simulink model "forced_choice"  (Simulink 6.6)
settings: Solver=FixedStepDiscrete  StartTime=0.0  StopTime=Inf  FixedStep=.001  RelTol=1e-3
undefined symbols (not defined in the file or in its folder): dfilt
libraries: xpclib x12, limblab x7, simulink x6, xpcnilib x4, dsparch4 x4, xpcmeasurementcomputinglib x2
CloseFcn:
  | rtwprivate ssgencode ModelCloseRequest rwalk_multi_local_v1
settings Model: Creator=limblab  LastModifiedBy=limblab  ExtModeArmWhenConnect=off  BufferReuse=off
settings DataIOCC: LimitDataPoints=off  SaveFormat=StructureWithTime  SaveState=on  SignalLoggingName=sigsOut
settings OptimizationCC: BlockReduction=off  BooleanDataType=off  OptimizeBlockIOStorage=off  BufferReuse=off  EnforceIntegerDowncast=off  ExpressionFolding=off  FoldNonRolledExpr=off  LocalBlockOutputs=off
settings DebuggingCC: SignalResolutionControl=TryResolveAllWithWarning  SolverPrmCheckMsg=none  MultiTaskDSMMsg=warning  MultiTaskCondExecSysMsg=none  StrictBusMsg=None
settings HardwareCC: TargetIntDivRoundTo=Floor  TargetEndianess=LittleEndian  TargetHWDeviceType=32-bit xPC Target (Intel Pentium)
settings RTWCC: SystemTargetFile=xpctarget.tlc  TemplateMakefile=xpc_default_tmf  Description=xPC Target  GenerateReport=on  ProcessScript=xpctarget_make_rtw_hook  IncludeERTFirstTime=on
settings xpcTargetCC: TargetFcnLib=ansi_tfl_tmw.mat  GenFloatMathFcnCalls=ANSI_C  PortableWordSizes=off

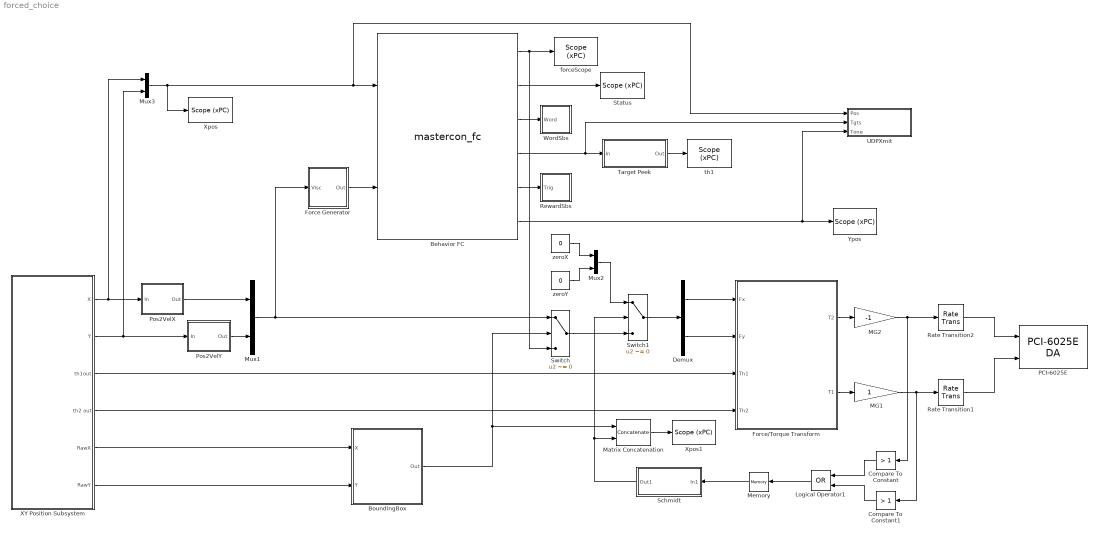
== system forced_choice ==
  Behavior FC : S-Function  FunctionName=mastercon_fc  Parameters=3 0 1 .5 1 .5 1 10 3 3 10
      mask Display:
      | disp('Master Control\nForced-Choice')
      | port_label('input',1,'pos')
      | port_label('input',2,'force')
      | port_label('output',1,'force')
      | port_label('output',2,'status')
      | port_label('output',3,'word')
      | port_label('output',4,'targets')
      | port_label('output',5,'reward')
      | port_label('output',6,'tone')
  BoundingBox : Subsystem
  Compare To Constant : simulink/Logic and Bit Operations/Compare To Constant  Orientation=left  SystemSampleTime=-1  relop=>  const=1  LogicOutDataTypeMode=uint8  ZeroCross=off
  Compare To Constant1 : simulink/Logic and Bit Operations/Compare To Constant  Orientation=left  SystemSampleTime=-1  relop=>  const=1  LogicOutDataTypeMode=uint8  ZeroCross=off
  Demux : Demux  Outputs=2
  Force Generator : Subsystem
  Force/Torque Transform : Subsystem  TreatAsAtomicUnit=on
      mask Display:
      | port_label('output', 1, 'T2')
      | port_label('output', 2, 'T1')
      | port_label('input', 1, 'Fx')
      | port_label('input', 2, 'Fy')
      | port_label('input', 3, 'Th1')
      | port_label('input', 4, 'Th2')
  Logical Operator1 : Logic  Orientation=left  Operator=OR  AllPortsSameDT=off  OutDataTypeMode=Boolean
  MG1 : Gain
  MG2 : Gain  Gain=-1
  Matrix Concatenation : Concatenate  Mode=Multidimensional array
  Memory : Memory  Orientation=left
  Mux1 : Mux  Inputs=2
  Mux2 : Mux  Inputs=2
  Mux3 : Mux  Inputs=2
  "PCI-6025E " : xpcnilib/D//A/PCI-6025E DA  channel=[1 2]  reset=[1 1]  initValue=[0 0]  sampletime=0.01  slot=[0 18]
  Pos2VelX : Subsystem
  Pos2VelY : Subsystem
  Rate Transition1 : RateTransition
  Rate Transition2 : RateTransition
  RewardSbs : Subsystem
  Schmidt : Subsystem  Orientation=left  mask(Schmidt Trigger){Time=10}
      mask help: Creates an output pulse of the specified time in seconds when trig goes high
      mask Help: Creates an output pulse of the specified time in seconds when trig goes high
      mask Display:
      | port_label('output',1,'out')
      | port_label('input',1,'trig')
      | fprintf('t = %d',Time)
  Status : xpclib/Misc./Scope (xPC)   SystemSampleTime=-1  scopeno=3  scopetype=Target  autostart=on  viewmode=Numerical  formatstr='%2.2f'  grid=on  ylimits=[-10,10]  nosamples=10  noprepostsamples=0  interleave=10  triggermode=FreeRun  triggersignal=1  triggerlevel=0.0  triggerslope=Either  triggerscope=1  triggersample=0  filename=data.dat  mode=Lazy  writesize=512  autorestart=off
  Switch : Switch  Criteria=u2 ~= 0  ZeroCross=off
  Switch1 : Switch  Criteria=u2 ~= 0  ZeroCross=off
  Target Peek : Subsystem
  UDPXmit : Subsystem
  WordSbs : Subsystem
  XY Position Subsystem : Subsystem
  Xpos : xpclib/Misc./Scope (xPC)   SystemSampleTime=-1  scopeno=1  scopetype=Target  autostart=on  viewmode=Numerical  formatstr=['%15.2f' '%15.2f']  grid=on  ylimits=[-10,10]  nosamples=10  noprepostsamples=0  interleave=10  triggermode=FreeRun  triggersignal=1  triggerlevel=0.0  triggerslope=Either  triggerscope=1  triggersample=0  filename=data.dat  mode=Lazy  writesize=512  autorestart=off
  Xpos1 : xpclib/Misc./Scope (xPC)   SystemSampleTime=-1  scopeno=5  scopetype=Target  autostart=on  viewmode=Numerical  formatstr='%15.2f'  grid=on  ylimits=[-10,10]  nosamples=10  noprepostsamples=0  interleave=10  triggermode=FreeRun  triggersignal=1  triggerlevel=0.0  triggerslope=Either  triggerscope=1  triggersample=0  filename=data.dat  mode=Lazy  writesize=512  autorestart=off
  Ypos : xpclib/Misc./Scope (xPC)   SystemSampleTime=-1  scopeno=2  scopetype=Target  autostart=on  viewmode=Numerical  formatstr='%15.2f'  grid=on  ylimits=[-10,10]  nosamples=10  noprepostsamples=0  interleave=10  triggermode=FreeRun  triggersignal=1  triggerlevel=0.0  triggerslope=Either  triggerscope=1  triggersample=0  filename=data.dat  mode=Lazy  writesize=512  autorestart=off
  forceScope : xpclib/Misc./Scope (xPC)   SystemSampleTime=-1  scopeno=7  scopetype=Target  autostart=on  viewmode=Numerical  formatstr='%2.2f'  grid=on  ylimits=[0,0]  nosamples=7  noprepostsamples=0  interleave=1  triggermode=FreeRun  triggersignal=1  triggerlevel=0.0  triggerslope=Either  triggerscope=1  triggersample=0  filename=data.dat  mode=Lazy  writesize=512  autorestart=off
  th1 : xpclib/Misc./Scope (xPC)   SystemSampleTime=-1  scopeno=4  scopetype=Target  autostart=on  viewmode=Numerical  formatstr=['%d' '%2.2f' '%2.2f']  grid=on  ylimits=[0,0]  nosamples=7  noprepostsamples=0  interleave=1  triggermode=FreeRun  triggersignal=1  triggerlevel=0.0  triggerslope=Either  triggerscope=1  triggersample=0  filename=data.dat  mode=Lazy  writesize=512  autorestart=off
  zeroX : Constant  Value=0
  zeroY : Constant  Value=0
  wires:
  XY Position Subsystem/1(X) -> Pos2VelX/1(In), Mux3/1
  XY Position Subsystem/2(Y) -> Pos2VelY/1(In), Mux3/2
  MG2/1 -> Rate Transition2/1, Compare To Constant/1
  MG1/1 -> Rate Transition1/1, Compare To Constant1/1
  Force/Torque Transform/1(T2) -> MG2/1
  Force/Torque Transform/2("T1 ") -> MG1/1
  XY Position Subsystem/3(th1out) -> Force/Torque Transform/3(Th1)
  XY Position Subsystem/4(th2 out) -> Force/Torque Transform/4(Th2)
  Demux/1 -> Force/Torque Transform/1(Fx)
  Demux/2 -> Force/Torque Transform/2(Fy)
  Mux1/1 -> Switch/1, Force Generator/1(Visc)
  XY Position Subsystem/5(RawX) -> BoundingBox/1(X)
  BoundingBox/1(Out) -> Switch/2, Matrix Concatenation/1
  zeroX/1 -> Mux2/1
  zeroY/1 -> Mux2/2
  Mux2/1 -> Switch1/1
  Rate Transition2/1 -> "PCI-6025E "/1
  Rate Transition1/1 -> "PCI-6025E "/2
  Switch/1 -> Switch1/3
  Switch1/1 -> Demux/1
  Schmidt/1(Out1) -> Switch1/2, Matrix Concatenation/2
  Compare To Constant/1 -> Logical Operator1/1
  Compare To Constant1/1 -> Logical Operator1/2
  Memory/1 -> Schmidt/1(In1)
  Logical Operator1/1 -> Memory/1
  Mux3/1 -> Xpos/1, Behavior FC/1, UDPXmit/1(Pos)
  Pos2VelX/1(Out) -> Mux1/1
  Pos2VelY/1(Out) -> Mux1/2
  XY Position Subsystem/6(RawY) -> BoundingBox/2(Y)
  Behavior FC/2 -> Status/1
  Behavior FC/3 -> WordSbs/1(Word)
  Behavior FC/4 -> Target Peek/1(In), UDPXmit/2(Tgts)
  Target Peek/1(Out) -> th1/1
  Behavior FC/6 -> UDPXmit/3(Tone), Ypos/1
  Force Generator/1(Out) -> Behavior FC/2
  Behavior FC/1 -> Switch/3, forceScope/1
  Matrix Concatenation/1 -> Xpos1/1
  Behavior FC/5 -> RewardSbs/1(Trig)

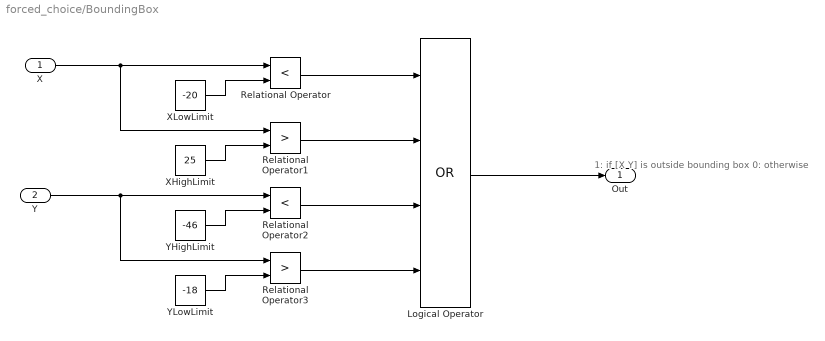
== system forced_choice/BoundingBox ==
  note: 1: if [X Y] is outside
      | bounding box
      | 0: otherwise
  X : Inport
  Y : Inport  Port=2
  Logical Operator : Logic  Operator=OR  Inputs=4  AllPortsSameDT=off  OutDataTypeMode=Boolean
  Relational Operator : RelationalOperator  Operator=<  LogicOutDataTypeMode=Boolean
  Relational Operator1 : RelationalOperator  Operator=>  LogicOutDataTypeMode=Boolean
  Relational Operator2 : RelationalOperator  Operator=<  LogicOutDataTypeMode=Boolean
  Relational Operator3 : RelationalOperator  Operator=>  LogicOutDataTypeMode=Boolean
  XHighLimit : Constant  Value=25
  XLowLimit : Constant  Value=-20
  YHighLimit : Constant  Value=-46
  YLowLimit : Constant  Value=-18
  Out : Outport
  wires:
  XLowLimit/1 -> Relational Operator/2
  XHighLimit/1 -> Relational Operator1/2
  YHighLimit/1 -> Relational Operator2/2
  YLowLimit/1 -> Relational Operator3/2
  Relational Operator/1 -> Logical Operator/1
  Relational Operator1/1 -> Logical Operator/2
  Relational Operator2/1 -> Logical Operator/3
  Relational Operator3/1 -> Logical Operator/4
  Logical Operator/1 -> Out/1
  X/1 -> Relational Operator/1, Relational Operator1/1
  Y/1 -> Relational Operator2/1, Relational Operator3/1

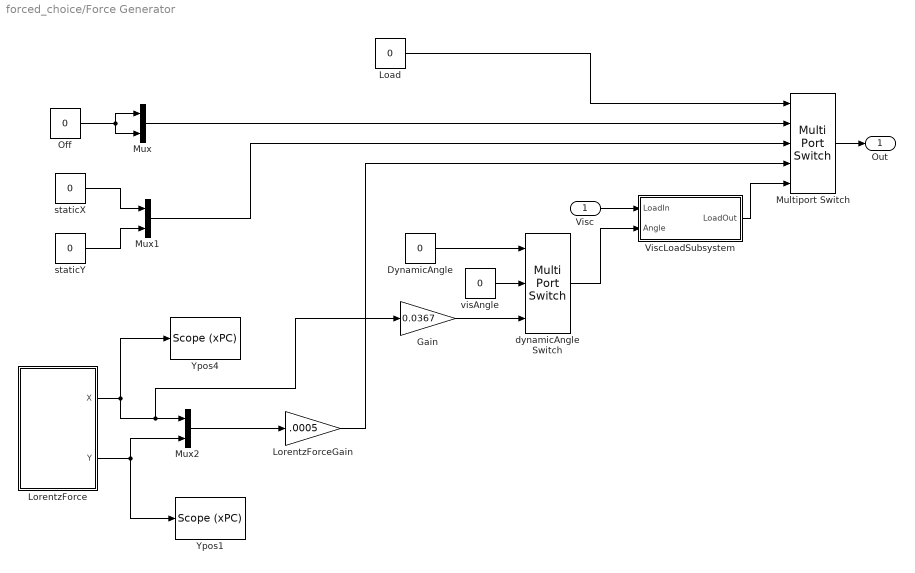
== system forced_choice/Force Generator ==
  Visc : Inport
  DynamicAngle : Constant  Value=0
  Gain : Gain  Gain=0.0367
  Load : Constant  Value=0
  LorentzForce : Subsystem
  LorentzForceGain : Gain  Gain=.0005
  Multiport Switch : MultiPortSwitch  zeroidx=on
  Mux : Mux  Inputs=2
  Mux1 : Mux  Inputs=2
  Mux2 : Mux  Inputs=2
  Off : Constant  Value=0
  ViscLoadSubsystem : Subsystem
  Ypos1 : xpclib/Misc./Scope (xPC)   SystemSampleTime=-1  scopeno=10  scopetype=Target  autostart=on  viewmode=Graphical rolling  formatstr='%15.2f'  grid=off  ylimits=[-30 30]  nosamples=200  noprepostsamples=0  interleave=10  triggermode=FreeRun  triggersignal=1  triggerlevel=0.0  triggerslope=Either  triggerscope=1  triggersample=0  filename=data.dat  mode=Lazy  writesize=512  autorestart=off
  Ypos4 : xpclib/Misc./Scope (xPC)   SystemSampleTime=-1  scopeno=9  scopetype=Target  autostart=on  viewmode=Graphical rolling  formatstr='%15.2f'  grid=on  ylimits=[-30 30]  nosamples=200  noprepostsamples=0  interleave=10  triggermode=FreeRun  triggersignal=1  triggerlevel=0.0  triggerslope=Either  triggerscope=1  triggersample=0  filename=data.dat  mode=Lazy  writesize=512  autorestart=off
  dynamicAngle Switch : MultiPortSwitch  Inputs=2  zeroidx=on
  staticX : Constant  Value=0
  staticY : Constant  Value=0
  visAngle : Constant  Value=0
  Out : Outport
  wires:
  Off/1 -> Mux/2, Mux/1
  Multiport Switch/1 -> Out/1
  Mux/1 -> Multiport Switch/2
  Load/1 -> Multiport Switch/1
  Mux1/1 -> Multiport Switch/3
  staticX/1 -> Mux1/1
  staticY/1 -> Mux1/2
  LorentzForce/1(X) -> Ypos4/1, Mux2/1, Gain/1
  LorentzForce/2(Y) -> Ypos1/1, Mux2/2
  Mux2/1 -> LorentzForceGain/1
  LorentzForceGain/1 -> Multiport Switch/4
  Visc/1 -> ViscLoadSubsystem/1(LoadIn)
  ViscLoadSubsystem/1(LoadOut) -> Multiport Switch/5
  visAngle/1 -> dynamicAngle Switch/2
  DynamicAngle/1 -> dynamicAngle Switch/1
  dynamicAngle Switch/1 -> ViscLoadSubsystem/2(Angle)
  Gain/1 -> dynamicAngle Switch/3

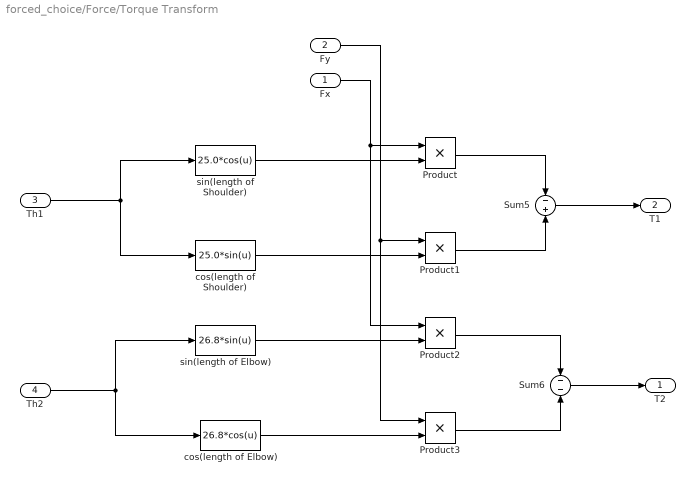
== system forced_choice/Force/Torque Transform ==
  Fx : Inport
  Fy : Inport  Port=2
  Th1 : Inport  Port=3
  Th2 : Inport  Port=4
  Product{,1..3} (4 alike) : Product  RndMeth=Zero
  Sum5 : Sum  Inputs=-+  SaturateOnIntegerOverflow=on  InputSameDT=on
  Sum6 : Sum  Inputs=--  SaturateOnIntegerOverflow=on  InputSameDT=on
  cos(length of Elbow) : Fcn  Expr=26.8*cos(u)
  cos(length of Shoulder) : Fcn  Expr=25.0*sin(u)
  sin(length of Elbow) : Fcn  Expr=26.8*sin(u)
  sin(length of Shoulder) : Fcn  Expr=25.0*cos(u)
  T2 : Outport
  "T1 " : Outport  Port=2
  wires:
  sin(length of Shoulder)/1 -> Product/2
  sin(length of Elbow)/1 -> Product2/2
  cos(length of Shoulder)/1 -> Product1/2
  cos(length of Elbow)/1 -> Product3/2
  Fx/1 -> Product/1, Product2/1
  Product/1 -> Sum5/1
  Fy/1 -> Product1/1, Product3/1
  Product1/1 -> Sum5/2
  Product2/1 -> Sum6/1
  Product3/1 -> Sum6/2
  Th1/1 -> sin(length of Shoulder)/1, cos(length of Shoulder)/1
  Th2/1 -> sin(length of Elbow)/1, cos(length of Elbow)/1
  Sum6/1 -> T2/1
  Sum5/1 -> "T1 "/1

== system forced_choice/Pos2VelX ==
  In : Inport
  Derivative : Derivative
  Digital Filter : dsparch4/Digital Filter  DialogController=dspdialog.DigitalFilter  DialogControllerArgs=DataTag0  TypePopup=FIR (all zeros)  IIRFiltStruct=Direct form II transposed  AllPoleFiltStruct=Direct form  FIRFiltStruct=Direct form  CoeffSource=Specify via dialog  NumCoeffs="[0.0144    0.0304    0.0724    0.1245    0.1668    0.1830    0.1668    0.1245    0.0724    0.0304    0.0144]"  DenCoeffs=[1 0.1]  BiQuadCoeffs=[1 0.3 0.4 1 0.1 0.2]  LatticeCoeffs=[0.2 0.4]  denIgnore=on  FiltPerSampPopup=One filter per frame  IC=0  ICnum=0  ICden=0  roundingMode=Floor  overflowMode=off  ScaleValues=1  scaleValueFracLength=14  stageInFracLength=15  stageOutFracLength=15  FilterSource=Specify via dialog  dfiltObjectName=dfilt.dffir([1 2 1])
  Digital Filter2 : dsparch4/Digital Filter  DialogController=dspdialog.DigitalFilter  DialogControllerArgs=DataTag1  TypePopup=FIR (all zeros)  IIRFiltStruct=Direct form II transposed  AllPoleFiltStruct=Direct form  FIRFiltStruct=Direct form  CoeffSource=Specify via dialog  NumCoeffs="[0.0144    0.0304    0.0724    0.1245    0.1668    0.1830    0.1668    0.1245    0.0724    0.0304    0.0144]"  DenCoeffs=[1 0.1]  BiQuadCoeffs=[1 0.3 0.4 1 0.1 0.2]  LatticeCoeffs=[0.2 0.4]  denIgnore=on  FiltPerSampPopup=One filter per frame  IC=0  ICnum=0  ICden=0  roundingMode=Floor  overflowMode=off  ScaleValues=1  scaleValueFracLength=14  stageInFracLength=15  stageOutFracLength=15  FilterSource=Specify via dialog  dfiltObjectName=dfilt.dffir([1 2 1])
  dG : Gain  Gain=-.0001  SampleTime=.001
  Out : Outport
  wires:
  Derivative/1 -> dG/1
  dG/1 -> Digital Filter/1
  Digital Filter2/1 -> Derivative/1
  In/1 -> Digital Filter2/1
  Digital Filter/1 -> Out/1

== system forced_choice/Pos2VelY ==
  In : Inport
  Derivative : Derivative
  Digital Filter : dsparch4/Digital Filter  DialogController=dspdialog.DigitalFilter  DialogControllerArgs=DataTag2  TypePopup=FIR (all zeros)  IIRFiltStruct=Direct form II transposed  AllPoleFiltStruct=Direct form  FIRFiltStruct=Direct form  CoeffSource=Specify via dialog  NumCoeffs="[0.0144    0.0304    0.0724    0.1245    0.1668    0.1830    0.1668    0.1245    0.0724    0.0304    0.0144]"  DenCoeffs=[1 0.1]  BiQuadCoeffs=[1 0.3 0.4 1 0.1 0.2]  LatticeCoeffs=[0.2 0.4]  denIgnore=on  FiltPerSampPopup=One filter per frame  IC=0  ICnum=0  ICden=0  roundingMode=Floor  overflowMode=off  ScaleValues=1  scaleValueFracLength=14  stageInFracLength=15  stageOutFracLength=15  FilterSource=Specify via dialog  dfiltObjectName=dfilt.dffir([1 2 1])
  Digital Filter2 : dsparch4/Digital Filter  DialogController=dspdialog.DigitalFilter  DialogControllerArgs=DataTag3  TypePopup=FIR (all zeros)  IIRFiltStruct=Direct form II transposed  AllPoleFiltStruct=Direct form  FIRFiltStruct=Direct form  CoeffSource=Specify via dialog  NumCoeffs="[0.0144    0.0304    0.0724    0.1245    0.1668    0.1830    0.1668    0.1245    0.0724    0.0304    0.0144]"  DenCoeffs=[1 0.1]  BiQuadCoeffs=[1 0.3 0.4 1 0.1 0.2]  LatticeCoeffs=[0.2 0.4]  denIgnore=on  FiltPerSampPopup=One filter per frame  IC=0  ICnum=0  ICden=0  roundingMode=Floor  overflowMode=off  ScaleValues=1  scaleValueFracLength=14  stageInFracLength=15  stageOutFracLength=15  FilterSource=Specify via dialog  dfiltObjectName=dfilt.dffir([1 2 1])
  dG : Gain  Gain=-.0001  SampleTime=.001
  Out : Outport
  wires:
  Derivative/1 -> dG/1
  dG/1 -> Digital Filter/1
  Digital Filter2/1 -> Derivative/1
  In/1 -> Digital Filter2/1
  Digital Filter/1 -> Out/1

== system forced_choice/RewardSbs ==
  Trig : Inport
  Data Type Conversion : DataTypeConversion
  Memory1 : Memory
  Schmidt1 : Subsystem  mask(Schmidt Trigger){Time=.3}
      mask help: Creates an output pulse of the specified time in seconds when trig goes high
      mask Help: Creates an output pulse of the specified time in seconds when trig goes high
      mask Display:
      | port_label('output',1,'out')
      | port_label('input',1,'trig')
      | fprintf('t = %.2f',Time)
  tag scope: Reward=global
  wires:
  Trig/1 -> Schmidt1/1(In1)
  Schmidt1/1(Out1) -> Memory1/1
  Memory1/1 -> Data Type Conversion/1
  Data Type Conversion/1 -> [Reward]

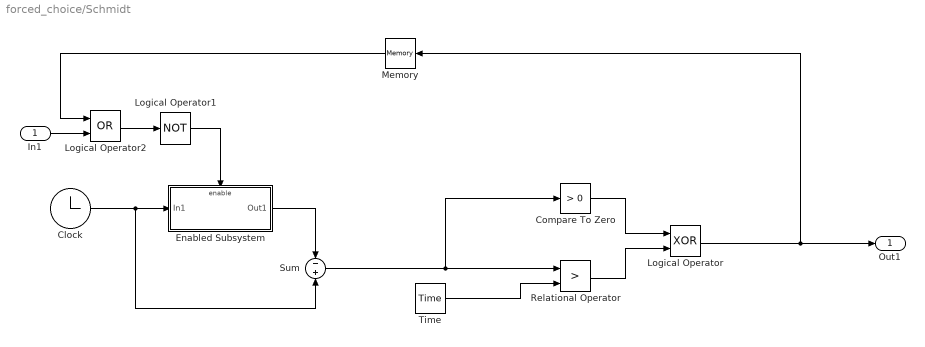
== system forced_choice/Schmidt ==
  In1 : Inport
  Clock : Clock
  Compare To Zero : simulink/Logic and Bit Operations/Compare To Zero  SystemSampleTime=-1  relop=>  LogicOutDataTypeMode=uint8  ZeroCross=off
  Enabled Subsystem : Subsystem  TreatAsAtomicUnit=on
  Logical Operator : Logic  Operator=XOR  AllPortsSameDT=off  OutDataTypeMode=Boolean  SampleTime=.001
  Logical Operator1 : Logic  Operator=NOT  AllPortsSameDT=off  OutDataTypeMode=Boolean
  Logical Operator2 : Logic  Operator=OR  AllPortsSameDT=off  OutDataTypeMode=Boolean  SampleTime=.001
  Memory : Memory  Orientation=left
  Relational Operator : RelationalOperator  Operator=>  LogicOutDataTypeMode=Boolean
  Sum : Sum  Inputs=-+
  Time : Constant  Value=Time
  Out1 : Outport
  wires:
  Clock/1 -> Enabled Subsystem/1(In1), Sum/2
  Enabled Subsystem/1(Out1) -> Sum/1
  Sum/1 -> Compare To Zero/1, Relational Operator/1
  Time/1 -> Relational Operator/2
  Compare To Zero/1 -> Logical Operator/1
  Relational Operator/1 -> Logical Operator/2
  Logical Operator1/1 -> Enabled Subsystem/Enable
  Logical Operator/1 -> Out1/1, Memory/1
  In1/1 -> Logical Operator2/2
  Logical Operator2/1 -> Logical Operator1/1
  Memory/1 -> Logical Operator2/1

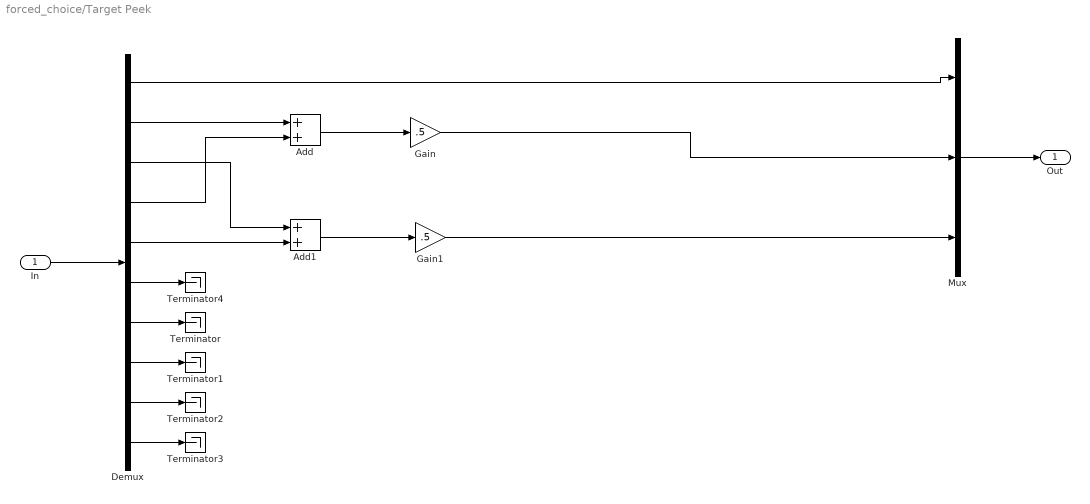
== system forced_choice/Target Peek ==
  In : Inport
  Add : Sum  OutScaling=2^-10
  Add1 : Sum  OutScaling=2^-10
  Demux : Demux  Outputs=10
  Gain : Gain  Gain=.5
  Gain1 : Gain  Gain=.5
  Mux : Mux  Inputs=3
  Terminator{,1..4} (5 alike) : Terminator
  Out : Outport
  wires:
  In/1 -> Demux/1
  Mux/1 -> Out/1
  Demux/1 -> Mux/1
  Add/1 -> Gain/1
  Add1/1 -> Gain1/1
  Gain1/1 -> Mux/3
  Demux/7 -> Terminator/1
  Demux/8 -> Terminator1/1
  Demux/9 -> Terminator2/1
  Demux/10 -> Terminator3/1
  Demux/2 -> Add/1
  Demux/4 -> Add/2
  Demux/3 -> Add1/1
  Demux/5 -> Add1/2
  Demux/6 -> Terminator4/1
  Gain/1 -> Mux/2

== system forced_choice/UDPXmit ==
  Pos : Inport
  Tgts : Inport  Port=2
  Tone : Inport  Port=3
  Demux : Demux  Outputs=10
  Demux1 : Demux  Outputs=2
  Demux2 : Demux  Outputs=2
  Pack : xpclib/UDP/Pack  datatypes={'double', 'double','double','double','double','double','double','double','double','double','double','double','double','double'}  byteAlign=1
  Rate Transition : RateTransition
  Send : xpclib/UDP/Send  ipAddress=192.168.0.2  ipPort=25000  localPort=-1  sampletime=.02
  wires:
  Rate Transition/1 -> Send/1
  Pack/1 -> Rate Transition/1
  Demux/10 -> Pack/12
  Demux/9 -> Pack/11
  Demux/8 -> Pack/10
  Demux/7 -> Pack/9
  Demux/6 -> Pack/8
  Demux/5 -> Pack/7
  Demux/4 -> Pack/6
  Demux/3 -> Pack/5
  Demux/2 -> Pack/4
  Demux/1 -> Pack/3
  Demux1/1 -> Pack/1
  Demux1/2 -> Pack/2
  Pos/1 -> Demux1/1
  Tgts/1 -> Demux/1
  Tone/1 -> Demux2/1
  Demux2/1 -> Pack/13
  Demux2/2 -> Pack/14

== system forced_choice/WordSbs ==
  Word : Inport
  Port A : xpcnilib/Digital Output/PCI-6025E 8255 DO  channel=1:8  port=A  reset=[1]  initValue=[0]  chip=1  sampletime=-1  slot=[0 16]
  ToBits : limblab/ToBits
  wires:
  Word/1 -> ToBits/1
  ToBits/1 -> Port A/1
  ToBits/2 -> Port A/2
  ToBits/3 -> Port A/3
  ToBits/4 -> Port A/4
  ToBits/5 -> Port A/5
  ToBits/6 -> Port A/6
  ToBits/7 -> Port A/7
  ToBits/8 -> Port A/8

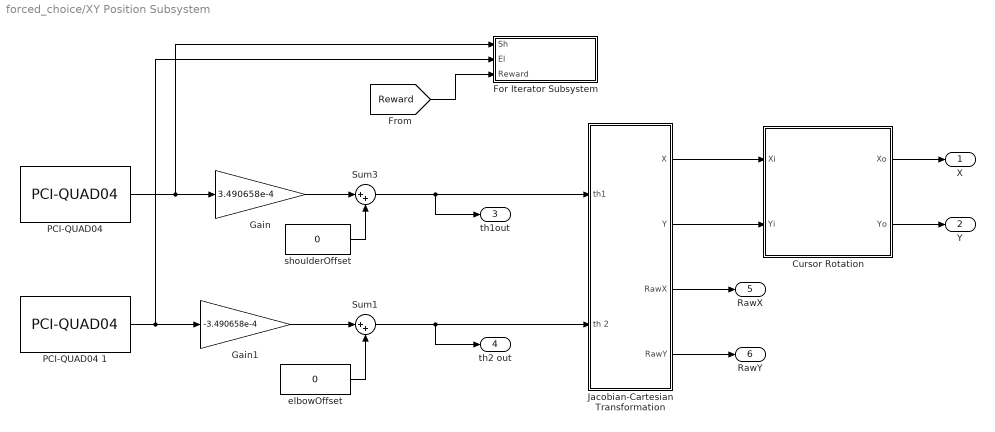
== system forced_choice/XY Position Subsystem ==
  Cursor Rotation : Subsystem
  For Iterator Subsystem : Subsystem  TreatAsAtomicUnit=on
  Gain : Gain  Gain=3.490658e-4
  Gain1 : Gain  Gain=-3.490658e-4
  Jacobian-Cartesian Transformation : Subsystem
  "PCI-QUAD04 " : xpcmeasurementcomputinglib/Incremental Encoder/PCI-QUAD04   channel=1  resetmode=on  polarity=Positive Index  mode=Normal  limit=0  range=-2^23...+2^23-1  speed=1x  prescale=0  ts=0.001  convbaseaddr=-1
  PCI-QUAD04 1 : xpcmeasurementcomputinglib/Incremental Encoder/PCI-QUAD04   channel=2  resetmode=on  polarity=Positive Index  mode=Normal  limit=0  range=-2^23...+2^23-1  speed=1x  prescale=0  ts=0.001  convbaseaddr=-1
  Sum1 : Sum  Inputs=|++  SaturateOnIntegerOverflow=on  InputSameDT=on
  Sum3 : Sum  Inputs=|++  SaturateOnIntegerOverflow=on  InputSameDT=on
  elbowOffset : Constant  Value=0
  shoulderOffset : Constant  Value=0
  X : Outport
  Y : Outport  Port=2
  th1out : Outport  Port=3
  th2 out : Outport  Port=4
  RawX : Outport  Port=5
  RawY : Outport  Port=6
  wires:
  PCI-QUAD04 1/1 -> Gain1/1, For Iterator Subsystem/2("El ")
  "PCI-QUAD04 "/1 -> Gain/1, For Iterator Subsystem/1(Sh)
  Gain/1 -> Sum3/1
  Sum3/1 -> Jacobian-Cartesian Transformation/1(th1), th1out/1
  shoulderOffset/1 -> Sum3/2
  Gain1/1 -> Sum1/1
  elbowOffset/1 -> Sum1/2
  Sum1/1 -> Jacobian-Cartesian Transformation/2(th 2), th2 out/1
  Jacobian-Cartesian Transformation/1(X) -> Cursor Rotation/1(Xi)
  Jacobian-Cartesian Transformation/2(Y) -> Cursor Rotation/2(Yi)
  Cursor Rotation/1(Xo) -> X/1
  Cursor Rotation/2(Yo) -> Y/1
  Jacobian-Cartesian Transformation/3(RawX) -> RawX/1
  Jacobian-Cartesian Transformation/4(RawY) -> RawY/1
  [Reward] -> For Iterator Subsystem/3(Reward)

== system forced_choice/Force Generator/LorentzForce ==
  Add : Sum  Inputs=+-  OutScaling=2^-10
  Add1 : Sum  Inputs=+-  OutScaling=2^-10
  Lorentz : limblab/Lorentz  SystemSampleTime=-1  y0=.1
  Lorentz1 : limblab/Lorentz  SystemSampleTime=-1  y0=.2
  Lorentz2 : limblab/Lorentz  SystemSampleTime=-1  y0=.3
  Lorentz3 : limblab/Lorentz  SystemSampleTime=-1  y0=.4
  X : Outport
  Y : Outport  Port=2
  wires:
  Lorentz/1 -> Add/1
  Lorentz1/1 -> Add/2
  Add/1 -> X/1
  Lorentz2/1 -> Add1/1
  Lorentz3/1 -> Add1/2
  Add1/1 -> Y/1

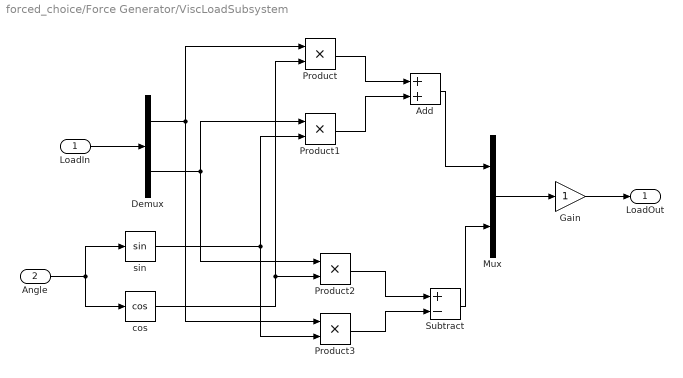
== system forced_choice/Force Generator/ViscLoadSubsystem ==
  LoadIn : Inport
  Angle : Inport  Port=2
  Add : Sum  OutScaling=2^-10
  Demux : Demux  Outputs=2
  Gain : Gain
  Mux : Mux  Inputs=2
  Product{,1..3} (4 alike) : Product  RndMeth=Zero
  Subtract : Sum  Inputs=+-  OutScaling=2^-10
  cos : Trigonometry  Operator=cos
  sin : Trigonometry
  LoadOut : Outport
  wires:
  LoadIn/1 -> Demux/1
  Mux/1 -> Gain/1
  Gain/1 -> LoadOut/1
  Angle/1 -> sin/1, cos/1
  Add/1 -> Mux/1
  Subtract/1 -> Mux/2
  Product/1 -> Add/1
  Product1/1 -> Add/2
  Product2/1 -> Subtract/1
  Product3/1 -> Subtract/2
  Demux/1 -> Product/1, Product3/1
  cos/1 -> Product/2, Product2/2
  Demux/2 -> Product1/1, Product2/1
  sin/1 -> Product1/2, Product3/2

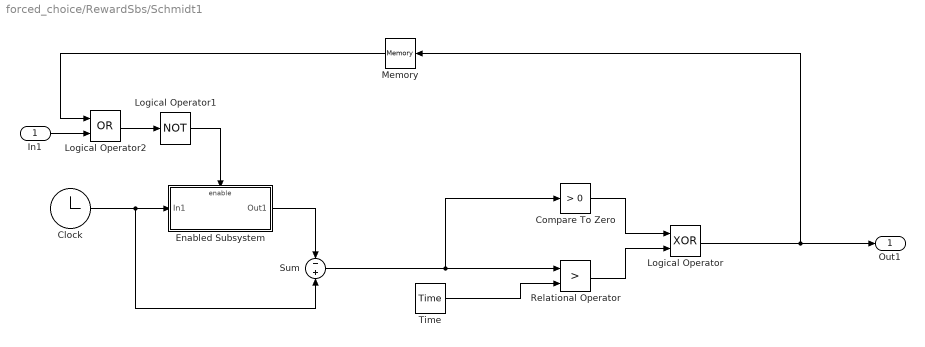
== system forced_choice/RewardSbs/Schmidt1 ==
  In1 : Inport
  Clock : Clock
  Compare To Zero : simulink/Logic and Bit Operations/Compare To Zero  SystemSampleTime=-1  relop=>  LogicOutDataTypeMode=uint8  ZeroCross=off
  Enabled Subsystem : Subsystem  TreatAsAtomicUnit=on
  Logical Operator : Logic  Operator=XOR  AllPortsSameDT=off  OutDataTypeMode=Boolean  SampleTime=.001
  Logical Operator1 : Logic  Operator=NOT  AllPortsSameDT=off  OutDataTypeMode=Boolean
  Logical Operator2 : Logic  Operator=OR  AllPortsSameDT=off  OutDataTypeMode=Boolean  SampleTime=.001
  Memory : Memory  Orientation=left
  Relational Operator : RelationalOperator  Operator=>  LogicOutDataTypeMode=Boolean
  Sum : Sum  Inputs=-+
  Time : Constant  Value=Time
  Out1 : Outport
  wires:
  Clock/1 -> Enabled Subsystem/1(In1), Sum/2
  Enabled Subsystem/1(Out1) -> Sum/1
  Sum/1 -> Compare To Zero/1, Relational Operator/1
  Time/1 -> Relational Operator/2
  Compare To Zero/1 -> Logical Operator/1
  Relational Operator/1 -> Logical Operator/2
  Logical Operator1/1 -> Enabled Subsystem/Enable
  Logical Operator/1 -> Out1/1, Memory/1
  In1/1 -> Logical Operator2/2
  Logical Operator2/1 -> Logical Operator1/1
  Memory/1 -> Logical Operator2/1

== system forced_choice/Schmidt/Enabled Subsystem ==
  In1 : Inport
  Enable : EnablePort
  Out1 : Outport
  wires:
  In1/1 -> Out1/1

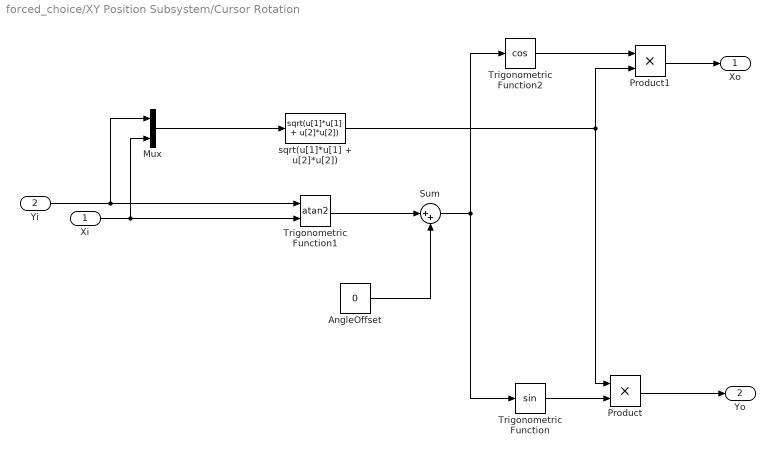
== system forced_choice/XY Position Subsystem/Cursor Rotation ==
  Xi : Inport
  Yi : Inport  Port=2
  AngleOffset : Constant  Value=0  SampleTime=.001
  Mux : Mux  Inputs=2
  Product : Product  RndMeth=Zero
  Product1 : Product  RndMeth=Zero
  Sum : Sum  Inputs=|++
  Trigonometric Function : Trigonometry
  Trigonometric Function1 : Trigonometry  Operator=atan2
  Trigonometric Function2 : Trigonometry  Operator=cos
  sqrt(u[1]*u[1] + u[2]*u[2]) : Fcn  Expr=sqrt(u[1]*u[1] + u[2]*u[2])
  Xo : Outport
  Yo : Outport  Port=2
  wires:
  AngleOffset/1 -> Sum/2
  Trigonometric Function1/1 -> Sum/1
  Yi/1 -> Trigonometric Function1/1, Mux/1
  Xi/1 -> Trigonometric Function1/2, Mux/2
  Mux/1 -> sqrt(u[1]*u[1] + u[2]*u[2])/1
  Trigonometric Function/1 -> Product/2
  Product/1 -> Yo/1
  sqrt(u[1]*u[1] + u[2]*u[2])/1 -> Product/1, Product1/2
  Sum/1 -> Trigonometric Function/1, Trigonometric Function2/1
  Product1/1 -> Xo/1
  Trigonometric Function2/1 -> Product1/1

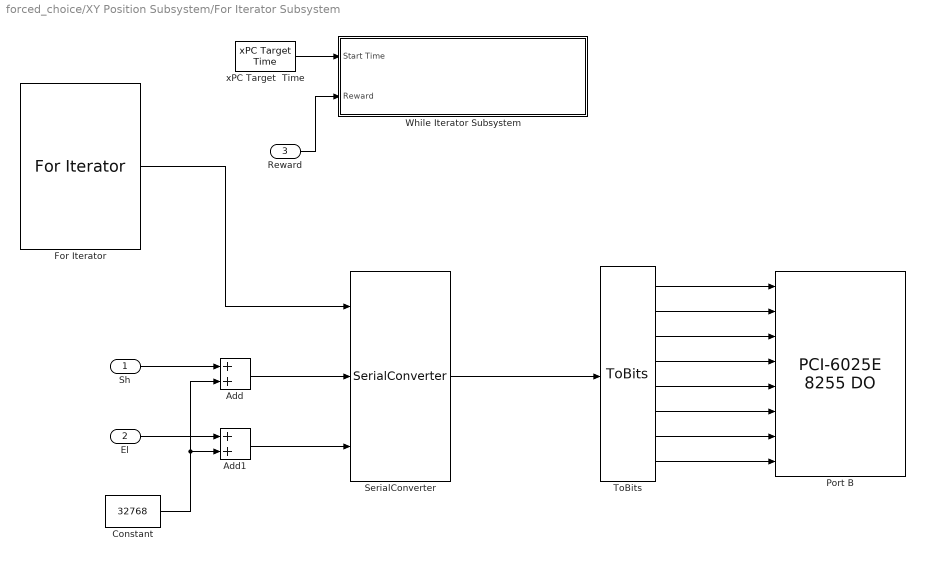
== system forced_choice/XY Position Subsystem/For Iterator Subsystem ==
  Sh : Inport
  "El " : Inport  Port=2
  Reward : Inport  Port=3
  Add : Sum  OutScaling=2^-10
  Add1 : Sum  OutScaling=2^-10
  Constant : Constant  Value=32768
  For Iterator : ForIterator  IterationLimit=4  IndexMode=Zero-based  IterationVariableDataType=double
  Port B : xpcnilib/Digital Output/PCI-6025E 8255 DO  channel=1:8  port=B  reset=[1]  initValue=[0]  chip=1  sampletime=-1  slot=[0 16]
  SerialConverter : limblab/SerialConverter
  ToBits : limblab/ToBits
  While Iterator Subsystem : Subsystem  TreatAsAtomicUnit=on
  "xPC Target  Time " : xpclib/Misc./xPC Target  Time   ts=-1
  wires:
  "xPC Target  Time "/1 -> While Iterator Subsystem/1(Start Time)
  SerialConverter/1 -> ToBits/1
  For Iterator/1 -> SerialConverter/1
  Sh/1 -> Add/1
  Add/1 -> SerialConverter/2
  Add1/1 -> SerialConverter/3
  "El "/1 -> Add1/1
  Constant/1 -> Add/2, Add1/2
  ToBits/1 -> Port B/1
  ToBits/2 -> Port B/2
  ToBits/3 -> Port B/3
  ToBits/4 -> Port B/4
  ToBits/5 -> Port B/5
  ToBits/6 -> Port B/6
  ToBits/7 -> Port B/7
  ToBits/8 -> Port B/8
  Reward/1 -> While Iterator Subsystem/2(Reward)

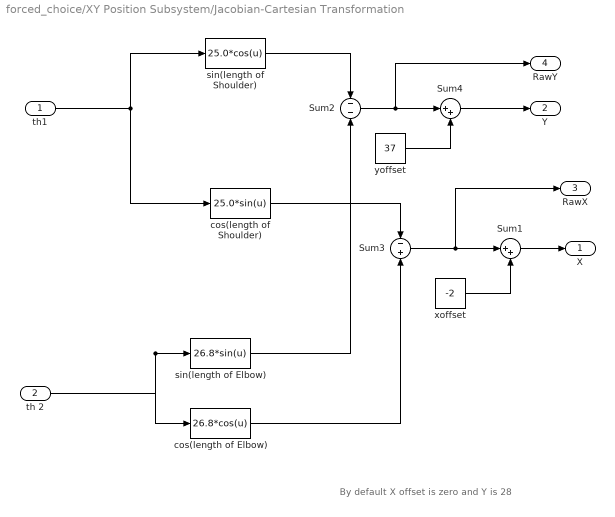
== system forced_choice/XY Position Subsystem/Jacobian-Cartesian Transformation ==
  note: By default X offset is zero and Y is 28
  th1 : Inport
  th 2 : Inport  Port=2
  Sum1 : Sum  Inputs=|++  SaturateOnIntegerOverflow=on  InputSameDT=on
  Sum2 : Sum  Inputs=--  SaturateOnIntegerOverflow=on  InputSameDT=on
  Sum3 : Sum  Inputs=-+  SaturateOnIntegerOverflow=on  InputSameDT=on
  Sum4 : Sum  Inputs=|++  SaturateOnIntegerOverflow=on  InputSameDT=on
  cos(length of Elbow) : Fcn  Expr=26.8*cos(u)
  cos(length of Shoulder) : Fcn  Expr=25.0*sin(u)
  sin(length of Elbow) : Fcn  Expr=26.8*sin(u)
  sin(length of Shoulder) : Fcn  Expr=25.0*cos(u)
  xoffset : Constant  Value=-2
  yoffset : Constant  Value=37
  X : Outport
  Y : Outport  Port=2
  RawX : Outport  Port=3
  RawY : Outport  Port=4
  wires:
  th1/1 -> sin(length of Shoulder)/1, cos(length of Shoulder)/1
  sin(length of Shoulder)/1 -> Sum2/1
  sin(length of Elbow)/1 -> Sum2/2
  Sum3/1 -> Sum1/1, RawX/1
  cos(length of Shoulder)/1 -> Sum3/1
  th 2/1 -> sin(length of Elbow)/1, cos(length of Elbow)/1
  Sum2/1 -> Sum4/1, RawY/1
  Sum4/1 -> Y/1
  Sum1/1 -> X/1
  xoffset/1 -> Sum1/2
  yoffset/1 -> Sum4/2
  cos(length of Elbow)/1 -> Sum3/2

== system forced_choice/RewardSbs/Schmidt1/Enabled Subsystem ==
  In1 : Inport
  Enable : EnablePort
  Out1 : Outport
  wires:
  In1/1 -> Out1/1

== system forced_choice/XY Position Subsystem/For Iterator Subsystem/While Iterator Subsystem ==
  Start Time : Inport
  Reward : Inport  Port=2
  Compare To Constant : simulink/Logic and Bit Operations/Compare To Constant  SystemSampleTime=-1  relop=<=  const=100  LogicOutDataTypeMode=boolean
  Compare To Constant1 : simulink/Logic and Bit Operations/Compare To Constant  SystemSampleTime=-1  relop=>  const=50  LogicOutDataTypeMode=boolean  ZeroCross=off
  Constant : Constant
  Constant1 : Constant  Value=0
  "PCI-6025E " : xpcnilib/Digital Output/PCI-6025E DO  channel=[1 2]  reset=[1]  initValue=[0]  sampletime=-1  slot=[0 16]
  ScaleTouSec : Gain  Gain=.838
  Subtract : Sum  Inputs=+-  OutScaling=2^-10
  Switch : Switch  Criteria=u2 ~= 0
  While Iterator : WhileIterator  MaxIters=-1  WhileBlockType=do-while
  "xPC Target  Time " : xpclib/Misc./xPC Target  Time   ts=-1
  wires:
  "xPC Target  Time "/1 -> Subtract/1
  Start Time/1 -> Subtract/2
  Subtract/1 -> ScaleTouSec/1
  Compare To Constant/1 -> While Iterator/1
  ScaleTouSec/1 -> Compare To Constant/1, Compare To Constant1/1
  Compare To Constant1/1 -> Switch/2
  Constant/1 -> Switch/1
  Constant1/1 -> Switch/3
  Switch/1 -> "PCI-6025E "/1
  Reward/1 -> "PCI-6025E "/2
